simulink model "DP_CFGOC_SSP"  (R2023b)
settings: Solver=ode45  StartTime=0.0  StopTime=300  RelTol=1e-3  EnableMultiTasking=on
undefined symbols (not defined in the file): Als, Ats, D, G, Loa, MA, MRB, pa, Ta_p, Ta_x, Ta_y
libraries: mssSimulink x8, simulink x8, simulink_extras x5, fuzblock x3, marine_gnc x3
settings Model: Creator=Lenovo  LastModifiedBy=Ly Soi
settings SolverCC: AlgebraicLoopSolver=TrustRegion
settings DataIOCC: LimitDataPoints=on  SaveFormat=Array  SignalLoggingSaveFormat=ModelDataLogs  ReturnWorkspaceOutputs=off  SignalLoggingName=sigsOut
settings OptimizationCC: InitFltsAndDblsToZero=on  LifeSpan=inf
settings DebuggingCC: SaveWithParameterizedLinksMsg=none  UnderspecifiedInitializationDetection=Classic  MergeDetectMultiDrivingBlocksExec=none  SignalResolutionControl=TryResolveAllWithWarning  MultiTaskDSMMsg=warning  MultiTaskCondExecSysMsg=none  FcnCallInpInsideContextMsg=warning  UnconnectedInputMsg=warning  UnconnectedOutputMsg=warning  UnconnectedLineMsg=warning  SFUnexpectedBacktrackingDiag=warning  SFNoUnconditionalDefaultTransitionDiag=warning  ArithmeticOperatorsInVariantConditions=warning
settings HardwareCC: ProdBitPerPointer=32  ProdBitPerSizeT=32  ProdBitPerPtrDiffT=32  ProdLargestAtomicFloat=None  ProdIntDivRoundTo=Undefined  ProdEndianess=Unspecified  ProdWordSize=32  ProdHWDeviceType=32-bit Generic  TargetUnknown=on
settings ModelReferenceCC: EnableRefExpFcnMdlSchedulingChecks=on  PropagateSignalLabelsOutOfModel=off
settings SFSimCC: SimUseLocalCustomCode=off  CustomCodeUndefinedFunction=UseInterfaceOnly
settings RTWCC: RTWUseLocalCustomCode=off
settings CodeAppCC: StateflowObjectComments=on
settings GRTTargetCC: TargetFcnLib=ansi_tfl_tmw.mat  TargetLangStandard=C89/C90 (ANSI)  ModelReferenceCompliant=off  CombineOutputUpdateFcns=off  MatFileLogging=off  GRTInterface=on
settings ConfigComp: CovMetricSettings=dw  CovSaveCumulativeToWorkspaceVar=on  CovSaveSingleToWorkspaceVar=on  CovExternalEMLEnable=off  CovSFcnEnable=off

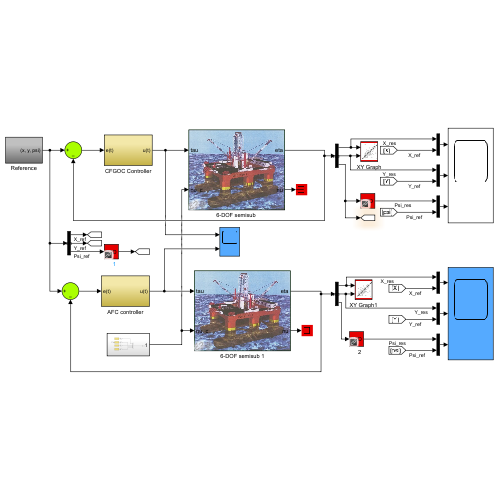
[thumbnail: Simulink's stored preview of the top-level diagram]
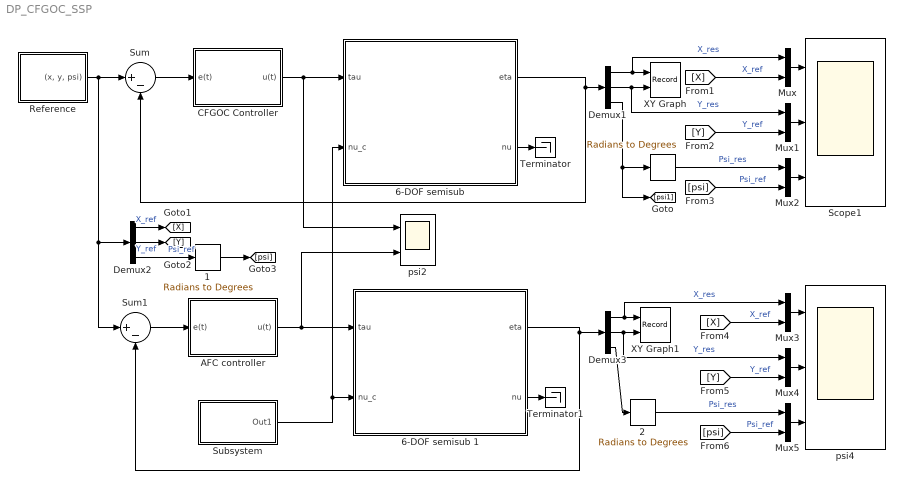
== system DP_CFGOC_SSP ==
  "    " : simulink_extras/Transformations/Radians to Degrees
  "    1" : simulink_extras/Transformations/Radians to Degrees
  "    2" : simulink_extras/Transformations/Radians to Degrees
  "6-DOF semisub " : Subsystem  AncestorBlock=mssSimulink/Marine craft models/6-DOF semisub  InitFcn=load MSS/VESSELS/rigModel/rig.mat  mask(6-DOF semisub){D=D, G=G, MA=MA, MRB=MRB}
      mask prompts: D "Linear damping matrix: D"; G "Spring matrix G:"; MA "System inertia added mass matrix: M"; MRB "System inertia rigid-body matrix"
      mask help:
      | Semisub low-speed model for DP.
      |
      | Inputs:
      |
      |    tau = 6 DOF control input vector (generalized force)
      |
      | Outputs:
      |
      |    eta = [x, y, z, phi, theta, psi]'
      |    nu  = [u, v, w, p, q, r]'
      mask Display:
      | image(imread('SIMULINK/figs/semisub.jpg'))
      | color('black'); port_label('output', 1, 'eta')
      | color('black'); port_label('output', 2, 'nu')
      | color('black'); port_label('input', 1, 'tau')
      | color('black'); port_label('input', 2, 'nu_c')
  6-DOF semisub 1 : Subsystem  AncestorBlock=mssSimulink/Marine craft models/6-DOF semisub  InitFcn=load MSS/VESSELS/rigModel/rig.mat  mask(6-DOF semisub){D=D, G=G, MA=MA, MRB=MRB}
      mask prompts: D "Linear damping matrix: D"; G "Spring matrix G:"; MA "System inertia added mass matrix: M"; MRB "System inertia rigid-body matrix"
      mask help:
      | Semisub low-speed model for DP.
      |
      | Inputs:
      |
      |    tau = 6 DOF control input vector (generalized force)
      |
      | Outputs:
      |
      |    eta = [x, y, z, phi, theta, psi]'
      |    nu  = [u, v, w, p, q, r]'
      mask Display:
      | image(imread('SIMULINK/figs/semisub.jpg'))
      | color('black'); port_label('output', 1, 'eta')
      | color('black'); port_label('output', 2, 'nu')
      | color('black'); port_label('input', 1, 'tau')
      | color('black'); port_label('input', 2, 'nu_c')
  AFC controller : Subsystem
  CFGOC Controller : Subsystem
  Demux1 : Demux  Outputs=3
      settings: DisplayOption=none
  Demux2 : Demux  Outputs=3
      settings: DisplayOption=none
  Demux3 : Demux  Outputs=3
      settings: DisplayOption=none
  Mux{,1..5} (6 alike) : Mux  Inputs=2
  Reference : Subsystem
  Scope1 : Scope  NumInputPorts=3
  Subsystem : Subsystem
  Sum : Sum  Inputs=|+-
  Sum1 : Sum  Inputs=|+-
  Terminator : Terminator
  Terminator1 : Terminator
  XY Graph : Record  FileSettingsInternal="{\"entries\":[{\"content\":{\"excelSettings\":{\"content\":{},\"type\":\"Streamout.ExcelSettings\"}},\"type\":\"Streamout.FileSettingStorage\",\"uuid\":\"\"}],\"packageUris\":[\"http:\\/\\/schema.mathworks.com\\/mf0\\/streamout_blocks\\/R2020a\"],\"version\":\"1.0\"}"  Layout=[1 1]  SignalsInternal="{\"entries\":[{\"content\":{\"signals\":[{\"content\":{\"blockPath\":[],\"dimensions\":[1],\"domain\":\"\",\"lineColor\":\"#a2142f\",\"plots\":[1],\"port\":1,\"signalID\":43,\"signalName\":\"XY Graph:1\"},\"type\":\"RecordBlkView.Signal\",\"uuid\":\"\"},{\"content\":{\"blockPath\":[],\"dimensions\":[1],\"domain\":\"\",\"lineColor\":\"#139fff\",\"plots\":[1],\"port\":2,\"signalID\":46,\"signalName\":\"XY Graph:2\"},\"type\":\"RecordBlkView.Signal\",\"uuid\":\"\"}]},\"type\":\"RecordBlkView.InputSignals\",\"uuid\":\"\"}],\"packageUris\":[\"http:\\/\\/schema.mathworks.com\\/mf0\\/streamout_blocks\\/R2020a\"],\"version\":\"1.0\"}"  VisualizationBindings="{\"xyplotplugin\":{\"info\":[{\"series\":[{\"bindingParametersList\":[{\"parameter\":\"X-Axis\",\"signalID\":43,\"signalName\":\"XY Graph:1\"},{\"parameter\":\"Y-Axis\",\"signalID\":46,\"signalName\":\"XY Graph:2\"}],\"seriesID\":58743}],\"subplotID\":1}]}}"  CompatibilityTag=XY  st=0.1
  XY Graph1 : Record  FileSettingsInternal="{\"entries\":[{\"content\":{\"excelSettings\":{\"content\":{},\"type\":\"Streamout.ExcelSettings\"}},\"type\":\"Streamout.FileSettingStorage\",\"uuid\":\"\"}],\"packageUris\":[\"http:\\/\\/schema.mathworks.com\\/mf0\\/streamout_blocks\\/R2020a\"],\"version\":\"1.0\"}"  Layout=[1 1]  SignalsInternal="{\"entries\":[{\"content\":{\"signals\":[{\"content\":{\"blockPath\":[],\"dimensions\":[1],\"domain\":\"\",\"lineColor\":\"#a2142f\",\"plots\":[1],\"port\":1,\"signalID\":35,\"signalName\":\"X_res\"},\"type\":\"RecordBlkView.Signal\",\"uuid\":\"\"},{\"content\":{\"blockPath\":[],\"dimensions\":[1],\"domain\":\"\",\"lineColor\":\"#139fff\",\"plots\":[1],\"port\":2,\"signalID\":38,\"signalName\":\"Y_res\"},\"type\":\"RecordBlkView.Signal\",\"uuid\":\"\"}]},\"type\":\"RecordBlkView.InputSignals\",\"uuid\":\"\"}],\"packageUris\":[\"http:\\/\\/schema.mathworks.com\\/mf0\\/streamout_blocks\\/R2020a\"],\"version\":\"1.0\"}"  VisualizationBindings="{\"xyplotplugin\":{\"info\":[{\"series\":[{\"bindingParametersList\":[{\"parameter\":\"X-Axis\",\"signalID\":35,\"signalName\":\"X_res\"},{\"parameter\":\"Y-Axis\",\"signalID\":38,\"signalName\":\"Y_res\"}],\"seriesID\":17634}],\"subplotID\":1}]}}"  CompatibilityTag=XY  st=0.1
  psi2 : Scope  NumInputPorts=2
  psi4 : Scope  NumInputPorts=3
  wires:
  Sum/1 -> CFGOC Controller/1(e(t))
  "6-DOF semisub "/2(nu) -> Terminator/1
  Demux1/1 -> XY Graph/1, Mux/1  "X_res"
  Demux1/2 -> XY Graph/2, Mux1/1  "Y_res"
  "6-DOF semisub "/1(eta) -> Sum/2, Demux1/1
  Demux1/3 -> "    "/1, [psi1]
  Mux/1 -> Scope1/1
  [X] -> Mux/2  "X_ref"
  Mux1/1 -> Scope1/2
  [Y] -> Mux1/2  "Y_ref"
  Mux2/1 -> Scope1/3
  [psi] -> Mux2/2  "Psi_ref"
  "    "/1 -> Mux2/1  "Psi_res"
  "    1"/1 -> [psi]
  Reference/1("(x, y, psi)") -> Sum1/1, Demux2/1, Sum/1
  Sum1/1 -> AFC controller/1(e(t))
  6-DOF semisub 1/2(nu) -> Terminator1/1
  Demux3/1 -> XY Graph1/1, Mux3/1  "X_res"
  Demux3/2 -> XY Graph1/2, Mux4/1  "Y_res"
  6-DOF semisub 1/1(eta) -> Sum1/2, Demux3/1
  Demux3/3 -> "    2"/1
  Mux3/1 -> psi4/1
  Demux2/1 -> [X]  "X_ref"
  Mux4/1 -> psi4/2
  Demux2/2 -> [Y]  "Y_ref"
  Mux5/1 -> psi4/3
  Demux2/3 -> "    1"/1  "Psi_ref"
  "    2"/1 -> Mux5/1  "Psi_res"
  [X] -> Mux3/2  "X_ref"
  [Y] -> Mux4/2  "Y_ref"
  [psi] -> Mux5/2  "Psi_ref"
  Subsystem/1(Out1) -> 6-DOF semisub 1/2(nu_c), "6-DOF semisub "/2(nu_c)
  CFGOC Controller/1(u(t)) -> psi2/1, "6-DOF semisub "/1(tau)
  AFC controller/1(u(t)) -> psi2/2, 6-DOF semisub 1/1(tau)

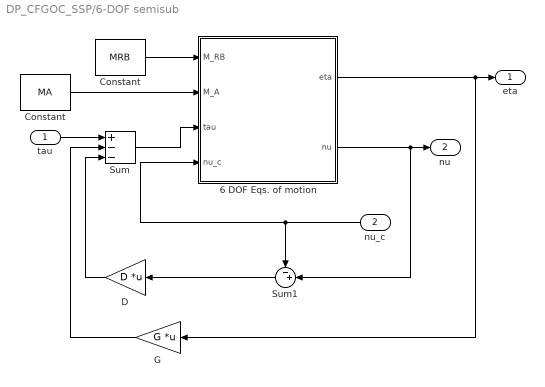
== system DP_CFGOC_SSP/6-DOF semisub  ==
  tau : Inport
  nu_c : Inport  Port=2
  "6 DOF Eqs. of motion " : Subsystem  AncestorBlock=mssSimulink/Modelling/Kinetics /6 DOF Eqs. of motion  mask(Equations of motion){CoriolisOnOff=on, nu0=[0 0 0 0 0 0], eta0=[0 0 0 0 0 0]}
      mask prompts: CoriolisOnOff "Coriolis and centripetal forces (check box to turn on)"; nu0 "Initial velocities (u,v,w,p,q,r)"; eta0 "Initial position/attitude (x,y,z,phi,theta,psi)"
      mask help:
      | 6 DOF equations of motion (surge, sway, heave, roll, pitch and yaw)
      |
      |    eta_dot = J(eta)*nu
      |    (M_RB+M_A)*nu_dot + C_RB(nu)nu+C_A(nu_r)nu_r  =  tau
      |
      |    nu_r = nu-nu_c    (relative velocity)
      |    nu_c = [u_c,v_c,w_c,0,0,0]  slowly-varying current velocity
      |
      | where nu = [u,v,w,p,q,r]'  and eta = [x,y,x,phi,theta,psi]'
      |
      | The Coriolis and centripetal matrix C(nu) is computed automatically using the system inertia matrix M and nu,  see Chapter 3 in Fossen (2002) for details.
      |
      | T. I. Fossen (2002). Marine Control Systems: Guidance, Navigation and Control of Ships, Rigs and Underwater Vehicles, Marine Cybernetics AS, ISBN 82-92356-00-2
  Constant : Constant  Value=MRB
  "Constant " : Constant  Value=MA
  D : Gain  Gain=D  Multiplication=Matrix(K*u)  SaturateOnIntegerOverflow=on  OutDataTypeStr=Inherit: Same as input  ParamDataTypeStr=Inherit: Same as input
  G : Gain  Gain=G  Multiplication=Matrix(K*u)  SaturateOnIntegerOverflow=on  OutDataTypeStr=Inherit: Same as input  ParamDataTypeStr=Inherit: Same as input
  Sum : Sum  Inputs=+--  InputSameDT=on  SaturateOnIntegerOverflow=on  OutDataTypeStr=Inherit: Same as first input
  Sum1 : Sum  Inputs=-+|  SaturateOnIntegerOverflow=on
  eta : Outport  InitialOutput=0  VectorParamsAs1DForOutWhenUnconnected=off
  nu : Outport  Port=2  InitialOutput=0  VectorParamsAs1DForOutWhenUnconnected=off
  wires:
  tau/1 -> Sum/1
  D/1 -> Sum/3
  G/1 -> Sum/2
  "6 DOF Eqs. of motion "/2(nu) -> Sum1/2, nu/1
  "6 DOF Eqs. of motion "/1(eta) -> eta/1, G/1
  Constant/1 -> "6 DOF Eqs. of motion "/1(M_RB)
  nu_c/1 -> Sum1/1, "6 DOF Eqs. of motion "/4(nu_c)
  Sum1/1 -> D/1
  Sum/1 -> "6 DOF Eqs. of motion "/3(tau)
  "Constant "/1 -> "6 DOF Eqs. of motion "/2(M_A)

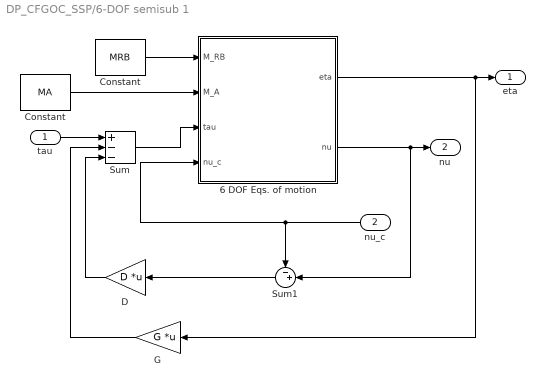
== system DP_CFGOC_SSP/6-DOF semisub 1 ==
  tau : Inport
  nu_c : Inport  Port=2
  "6 DOF Eqs. of motion " : Subsystem  AncestorBlock=mssSimulink/Modelling/Kinetics /6 DOF Eqs. of motion  mask(Equations of motion){CoriolisOnOff=on, nu0=[0 0 0 0 0 0], eta0=[0 0 0 0 0 0]}
      mask prompts: CoriolisOnOff "Coriolis and centripetal forces (check box to turn on)"; nu0 "Initial velocities (u,v,w,p,q,r)"; eta0 "Initial position/attitude (x,y,z,phi,theta,psi)"
      mask help:
      | 6 DOF equations of motion (surge, sway, heave, roll, pitch and yaw)
      |
      |    eta_dot = J(eta)*nu
      |    (M_RB+M_A)*nu_dot + C_RB(nu)nu+C_A(nu_r)nu_r  =  tau
      |
      |    nu_r = nu-nu_c    (relative velocity)
      |    nu_c = [u_c,v_c,w_c,0,0,0]  slowly-varying current velocity
      |
      | where nu = [u,v,w,p,q,r]'  and eta = [x,y,x,phi,theta,psi]'
      |
      | The Coriolis and centripetal matrix C(nu) is computed automatically using the system inertia matrix M and nu,  see Chapter 3 in Fossen (2002) for details.
      |
      | T. I. Fossen (2002). Marine Control Systems: Guidance, Navigation and Control of Ships, Rigs and Underwater Vehicles, Marine Cybernetics AS, ISBN 82-92356-00-2
  Constant : Constant  Value=MRB
  "Constant " : Constant  Value=MA
  D : Gain  Gain=D  Multiplication=Matrix(K*u)  SaturateOnIntegerOverflow=on  OutDataTypeStr=Inherit: Same as input  ParamDataTypeStr=Inherit: Same as input
  G : Gain  Gain=G  Multiplication=Matrix(K*u)  SaturateOnIntegerOverflow=on  OutDataTypeStr=Inherit: Same as input  ParamDataTypeStr=Inherit: Same as input
  Sum : Sum  Inputs=+--  InputSameDT=on  SaturateOnIntegerOverflow=on  OutDataTypeStr=Inherit: Same as first input
  Sum1 : Sum  Inputs=-+|  SaturateOnIntegerOverflow=on
  eta : Outport  InitialOutput=0  VectorParamsAs1DForOutWhenUnconnected=off
  nu : Outport  Port=2  InitialOutput=0  VectorParamsAs1DForOutWhenUnconnected=off
  wires:
  tau/1 -> Sum/1
  D/1 -> Sum/3
  G/1 -> Sum/2
  "6 DOF Eqs. of motion "/2(nu) -> Sum1/2, nu/1
  "6 DOF Eqs. of motion "/1(eta) -> eta/1, G/1
  Constant/1 -> "6 DOF Eqs. of motion "/1(M_RB)
  nu_c/1 -> Sum1/1, "6 DOF Eqs. of motion "/4(nu_c)
  Sum1/1 -> D/1
  Sum/1 -> "6 DOF Eqs. of motion "/3(tau)
  "Constant "/1 -> "6 DOF Eqs. of motion "/2(M_A)

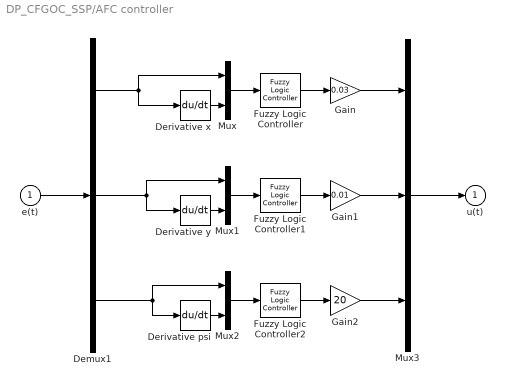
== system DP_CFGOC_SSP/AFC controller ==
  e(t) : Inport
  Demux1 : Demux  Outputs=3
  Derivative psi : Derivative
  Derivative x : Derivative
  Derivative y : Derivative
  Fuzzy Logic Controller : fuzblock/Fuzzy Logic  Controller  FIS='motau1moi.fis'  OutputSampleNumber=101  DataType=double  FuzzifiedInputs=off  RuleFiringStrengths=off  RuleOutputs=off  AggregatedOutputs=off  SimulateUsing=Interpreted execution  OutOfRangeInputValueMessage=warning  NoRuleFiredMessage=warning  EmptyOutputFuzzySetMessage=warning
  Fuzzy Logic Controller1 : fuzblock/Fuzzy Logic  Controller  FIS='motau2moi.fis'  OutputSampleNumber=101  DataType=double  FuzzifiedInputs=off  RuleFiringStrengths=off  RuleOutputs=off  AggregatedOutputs=off  SimulateUsing=Interpreted execution  OutOfRangeInputValueMessage=warning  NoRuleFiredMessage=warning  EmptyOutputFuzzySetMessage=warning
  Fuzzy Logic Controller2 : fuzblock/Fuzzy Logic  Controller  FIS='motau3moi.fis'  OutputSampleNumber=101  DataType=double  FuzzifiedInputs=off  RuleFiringStrengths=off  RuleOutputs=off  AggregatedOutputs=off  SimulateUsing=Interpreted execution  OutOfRangeInputValueMessage=warning  NoRuleFiredMessage=warning  EmptyOutputFuzzySetMessage=warning
  Gain : Gain  Gain=0.03
  Gain1 : Gain  Gain=0.01
  Gain2 : Gain  Gain=20
  Mux : Mux  Inputs=2
  Mux1 : Mux  Inputs=2
  Mux2 : Mux  Inputs=2
  Mux3 : Mux  Inputs=3
  u(t) : Outport
  wires:
  Mux3/1 -> u(t)/1
  e(t)/1 -> Demux1/1
  Gain1/1 -> Mux3/2
  Gain2/1 -> Mux3/3
  Fuzzy Logic Controller/1 -> Gain/1
  Gain/1 -> Mux3/1
  Fuzzy Logic Controller2/1 -> Gain2/1
  Fuzzy Logic Controller1/1 -> Gain1/1
  Demux1/1 -> Mux/1, Derivative x/1
  Demux1/2 -> Derivative y/1, Mux1/1
  Demux1/3 -> Derivative psi/1, Mux2/1
  Derivative y/1 -> Mux1/2
  Derivative x/1 -> Mux/2
  Derivative psi/1 -> Mux2/2
  Mux/1 -> Fuzzy Logic Controller/1
  Mux1/1 -> Fuzzy Logic Controller1/1
  Mux2/1 -> Fuzzy Logic Controller2/1

== system DP_CFGOC_SSP/CFGOC Controller ==
  e(t) : Inport
  Demux1 : Demux  Outputs=3
  GA-Psi : Subsystem
  GA-X : Subsystem
  GA-Y : Subsystem
  Gain : Gain  Gain=0.3
  Gain1 : Gain  Gain=0.3
  Gain2 : Gain
  Mux3 : Mux  Inputs=3
  u(t) : Outport
  wires:
  Mux3/1 -> u(t)/1
  Demux1/2 -> GA-Y/1(e_h)
  Demux1/3 -> GA-Psi/1(e_h)
  e(t)/1 -> Demux1/1
  Gain1/1 -> Mux3/2
  Gain2/1 -> Mux3/3
  GA-X/1(u_h) -> Gain/1
  Demux1/1 -> GA-X/1(e_h)
  Gain/1 -> Mux3/1
  GA-Psi/1(u_h) -> Gain2/1
  GA-Y/1(u_h) -> Gain1/1

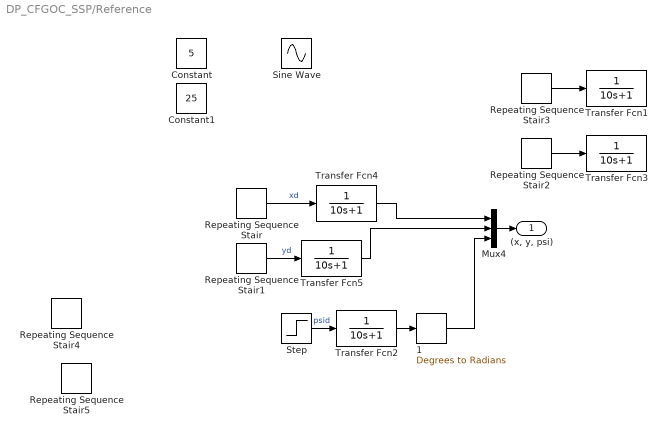
== system DP_CFGOC_SSP/Reference ==
  "     1" : simulink_extras/Transformations/Degrees to Radians
  Constant : Constant  Value=5
  Constant1 : Constant  Value=25
  Mux4 : Mux  Inputs=3
  Repeating Sequence Stair : simulink/Sources/Repeating Sequence Stair  OutValues=[10 0 10]  tsamp=100  OutMin=[]  OutMax=[]  OutDataTypeStr=double  OutputDataTypeScalingMode=double  OutDataType=fixdt(0,8)  ConRadixGroup=Best Precision: Vector-wise  OutScaling=2^-12
  Repeating Sequence Stair1 : simulink/Sources/Repeating Sequence Stair  OutValues=[0 10 10]  tsamp=100  OutMin=[]  OutMax=[]  OutDataTypeStr=double  OutputDataTypeScalingMode=double  OutDataType=fixdt(0,8)  ConRadixGroup=Best Precision: Vector-wise  OutScaling=2^-12
  Repeating Sequence Stair2 : simulink/Sources/Repeating Sequence Stair  OutValues=[7 -7 0 7]  tsamp=10  OutMin=[]  OutMax=[]  OutDataTypeStr=double  OutputDataTypeScalingMode=double  OutDataType=fixdt(0,8)  ConRadixGroup=Best Precision: Vector-wise  OutScaling=2^-12
  Repeating Sequence Stair3 : simulink/Sources/Repeating Sequence Stair  OutValues=[-7 7 0 7]  tsamp=10  OutMin=[]  OutMax=[]  OutDataTypeStr=double  OutputDataTypeScalingMode=double  OutDataType=fixdt(0,8)  ConRadixGroup=Best Precision: Vector-wise  OutScaling=2^-12
  Repeating Sequence Stair4 : simulink/Sources/Repeating Sequence Stair  OutValues="[0\t0\t0\t0\t0\t0\t0\t0\t0\t0\t0\t0\t0\t0\t0\t0\t0\t0\t0\t0\t0\t0\t0\t0\t0\t0\t0\t0\t0\t0\t0\t0\t0\t0\t0\t0\t0\t0\t0\t0\t0\t0\t0\t0\t0\t0\t0\t0\t0\t0\t0\t0\t0\t0\t0\t0\t0\t0\t0\t0\t0\t0\t0\t0\t0\t0\t0\t0\t0\t0\t0\t0\t0\t0\t0\t0\t0\t0\t0\t0\t0\t0\t0\t0\t0\t0\t0\t0\t0\t0\t0\t0\t0\t0\t0\t0\t0\t0\t0\t0\t0\t0\t0\t0.2\t0.4\t0.6\t0.8\t1\t1.2\t1.4\t1.6\t1.8\t2\t2.2\t2.4\t2.6\t2.8\t3\t3.2\t3.4\t3.6\t3.8\t4\t4.2\t4.4\t4.6\t4.8\t5\t5.2\t5.4\t5.6\t5.8\t6\t6.2\t6.4\t6.6\t6.8\t7\t7.2\t7.4\t7.6\t7.8\t8\t8.2\t8.4\t8.6\t8.8\t9\t9.2\t9.4\t9.6\t9.8\t10\t10\t10\t10\t10\t10\t10\t10\t10\t10\t10\t10\t10\t10\t10\t10\t10\t10\t10\t10\t10\t10\t10\t10\t10\t10\t10\t10\t10\t10\t10\t10\t10\t10\t10\t10\t10\t10\t10\t10\t10\t10\t10\t10\t10\t10\t10\t10\t10\t10\t10\t10]"  tsamp=1  OutMin=[]  OutMax=[]  OutDataTypeStr=double  OutputDataTypeScalingMode=double  OutDataType=fixdt(0,8)  ConRadixGroup=Best Precision: Vector-wise  OutScaling=2^-12
  Repeating Sequence Stair5 : simulink/Sources/Repeating Sequence Stair  OutValues="[0\t0.2\t0.4\t0.6\t0.8\t1\t1.2\t1.4\t1.6\t1.8\t2\t2.2\t2.4\t2.6\t2.8\t3\t3.2\t3.4\t3.6\t3.8\t4\t4.2\t4.4\t4.6\t4.8\t5\t5.2\t5.4\t5.6\t5.8\t6\t6.2\t6.4\t6.6\t6.8\t7\t7.2\t7.4\t7.6\t7.8\t8\t8.2\t8.4\t8.6\t8.8\t9\t9.2\t9.4\t9.6\t9.8\t10\t10\t10\t10\t10\t10\t10\t10\t10\t10\t10\t10\t10\t10\t10\t10\t10\t10\t10\t10\t10\t10\t10\t10\t10\t10\t10\t10\t10\t10\t10\t10\t10\t10\t10\t10\t10\t10\t10\t10\t10\t10\t10\t10\t10\t10\t10\t10\t10\t10\t10\t10\t10\t10\t10\t10\t10\t10\t10\t10\t10\t10\t10\t10\t10\t10\t10\t10\t10\t10\t10\t10\t10\t10\t10\t10\t10\t10\t10\t10\t10\t10\t10\t10\t10\t10\t10\t10\t10\t10\t10\t10\t10\t10\t10\t10\t10\t10\t10\t10\t10\t10\t10\t10\t10\t10\t10\t10\t10\t10\t10\t10\t10\t10\t10\t10\t10\t10\t10\t10\t10\t10\t10\t10\t10\t10\t10\t10\t10\t10\t10\t10\t10\t10\t10\t10\t10\t10\t10\t10\t10\t10\t10\t10\t10\t10\t10\t10\t10\t10\t10\t10\t10\t10]"  tsamp=1  OutMin=[]  OutMax=[]  OutDataTypeStr=double  OutputDataTypeScalingMode=double  OutDataType=fixdt(0,8)  ConRadixGroup=Best Precision: Vector-wise  OutScaling=2^-12
  Sine Wave : Sin  Frequency=4  SampleTime=0
  Step : Step  Time=0  After=20  SampleTime=0
  Transfer Fcn{1..5} (5 alike) : TransferFcn  Denominator=[10 1]
  "(x, y, psi)" : Outport
  wires:
  Mux4/1 -> "(x, y, psi)"/1
  "     1"/1 -> Mux4/3
  Step/1 -> Transfer Fcn2/1  "psid"
  Transfer Fcn2/1 -> "     1"/1
  Repeating Sequence Stair2/1 -> Transfer Fcn3/1
  Repeating Sequence Stair3/1 -> Transfer Fcn1/1
  Repeating Sequence Stair/1 -> Transfer Fcn4/1  "xd"
  Repeating Sequence Stair1/1 -> Transfer Fcn5/1  "yd"
  Transfer Fcn4/1 -> Mux4/1
  Transfer Fcn5/1 -> Mux4/2

== system DP_CFGOC_SSP/Subsystem ==
  Current impact : Subsystem
  Mux : Mux
  Noise impact : Subsystem
  Wave impact : Subsystem
  Wind impact : Subsystem
  adjust_Noi : Gain
  adjust_c : Gain
  adjust_w : Gain  Gain=2
  adjust_wi : Gain
  Out1 : Outport
  wires:
  Wave impact/1(Tau_wave) -> adjust_w/1
  Current impact/1(Tau_current) -> adjust_c/1
  [psi1] -> Wind impact/1(psi)
  Noise impact/1(Tau_Noise) -> adjust_Noi/1
  Wind impact/1(Tau_wind) -> adjust_wi/1
  adjust_wi/1 -> Mux/2
  adjust_w/1 -> Mux/1
  adjust_c/1 -> Mux/3
  adjust_Noi/1 -> Mux/4
  Mux/1 -> Out1/1

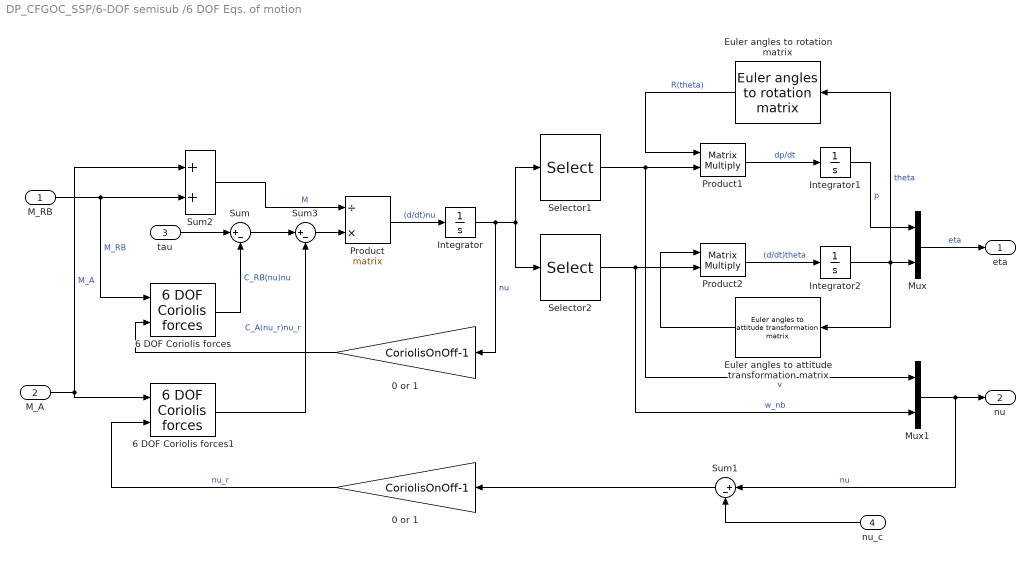
== system DP_CFGOC_SSP/6-DOF semisub /6 DOF Eqs. of motion  ==
  M_RB : Inport
  M_A : Inport  Port=2
  tau : Inport  Port=3
  nu_c : Inport  Port=4
  0 or 1 : Gain  Gain=CoriolisOnOff-1  SaturateOnIntegerOverflow=on  OutDataTypeStr=Inherit: Same as input  ParamDataTypeStr=Inherit: Same as input
  "0 or 1   " : Gain  Gain=CoriolisOnOff-1  SaturateOnIntegerOverflow=on  OutDataTypeStr=Inherit: Same as input  ParamDataTypeStr=Inherit: Same as input
  6 DOF Coriolis forces : mssSimulink/Modelling/Kinetics /Support/6 DOF Coriolis forces  SystemSampleTime=-1  VariantActivationTime=update diagram  AllowFlexibleInterface=on  Latency=0  AutoFrameSizeCalculation=off
  6 DOF Coriolis forces1 : mssSimulink/Modelling/Kinetics /Support/6 DOF Coriolis forces  SystemSampleTime=-1  VariantActivationTime=update diagram  AllowFlexibleInterface=on  Latency=0  AutoFrameSizeCalculation=off
  Euler angles to rotation matrix : mssSimulink/Modelling/Kinematics/Euler angles to rotation matrix
  Euler angles to attitude transformation matrix : mssSimulink/Modelling/Kinematics/Euler angles to attitude transformation matrix
  Integrator : Integrator  InitialCondition=nu0
  Integrator1 : Integrator  InitialCondition=eta0(1:3)
  Integrator2 : Integrator  InitialCondition=eta0(4:6)
  Mux : Mux  Inputs=2
  Mux1 : Mux  Inputs=2
  Product : Product  Inputs=/*  Multiplication=Matrix(*)  SaturateOnIntegerOverflow=on  OutDataTypeStr=Inherit: Same as first input
  Product1 : Product  Inputs=**  Multiplication=Matrix(*)  SaturateOnIntegerOverflow=on  OutDataTypeStr=Inherit: Same as first input
  Product2 : Product  Inputs=**  Multiplication=Matrix(*)  SaturateOnIntegerOverflow=on  OutDataTypeStr=Inherit: Same as first input
  Selector1 : Selector  InputPortWidth=6  IndexOptions=Index vector (dialog)  Indices=[1 2 3]  OutputSizes=1
  Selector2 : Selector  InputPortWidth=6  IndexOptions=Index vector (dialog)  Indices=[4 5 6]  OutputSizes=1
  Sum : Sum  Inputs=|+-  SaturateOnIntegerOverflow=on
  Sum1 : Sum  Inputs=|+-  SaturateOnIntegerOverflow=on
  Sum2 : Sum  SaturateOnIntegerOverflow=on
  Sum3 : Sum  Inputs=|+-  SaturateOnIntegerOverflow=on
  eta : Outport  VectorParamsAs1DForOutWhenUnconnected=off
  nu : Outport  Port=2  VectorParamsAs1DForOutWhenUnconnected=off
  wires:
  0 or 1/1 -> 6 DOF Coriolis forces/2
  6 DOF Coriolis forces/1 -> Sum/2  "C_RB(nu)nu"
  tau/1 -> Sum/1
  Euler angles to attitude transformation matrix/1 -> Product2/1
  Mux1/1 -> Sum1/1, nu/1  "nu"
  Mux/1 -> eta/1  "eta"
  Integrator1/1 -> Mux/1  "p"
  Integrator2/1 -> Euler angles to attitude transformation matrix/1, Euler angles to rotation matrix/1, Mux/2  "theta"
  Product2/1 -> Integrator2/1  "(d/dt)theta"
  Euler angles to rotation matrix/1 -> Product1/1  "R(theta)"
  Product1/1 -> Integrator1/1  "dp/dt"
  Selector2/1 -> Product2/2, Mux1/2  "w_nb"
  Selector1/1 -> Mux1/1, Product1/2  "v"
  Integrator/1 -> 0 or 1/1, Selector2/1, Selector1/1  "nu"
  Product/1 -> Integrator/1  "(d/dt)nu"
  M_RB/1 -> 6 DOF Coriolis forces/1, Sum2/2  "M_RB"
  M_A/1 -> 6 DOF Coriolis forces1/1, Sum2/1  "M_A"
  Sum2/1 -> Product/1  "M"
  Sum/1 -> Sum3/1
  Sum3/1 -> Product/2
  6 DOF Coriolis forces1/1 -> Sum3/2  "C_A(nu_r)nu_r"
  "0 or 1   "/1 -> 6 DOF Coriolis forces1/2  "nu_r"
  Sum1/1 -> "0 or 1   "/1
  nu_c/1 -> Sum1/2

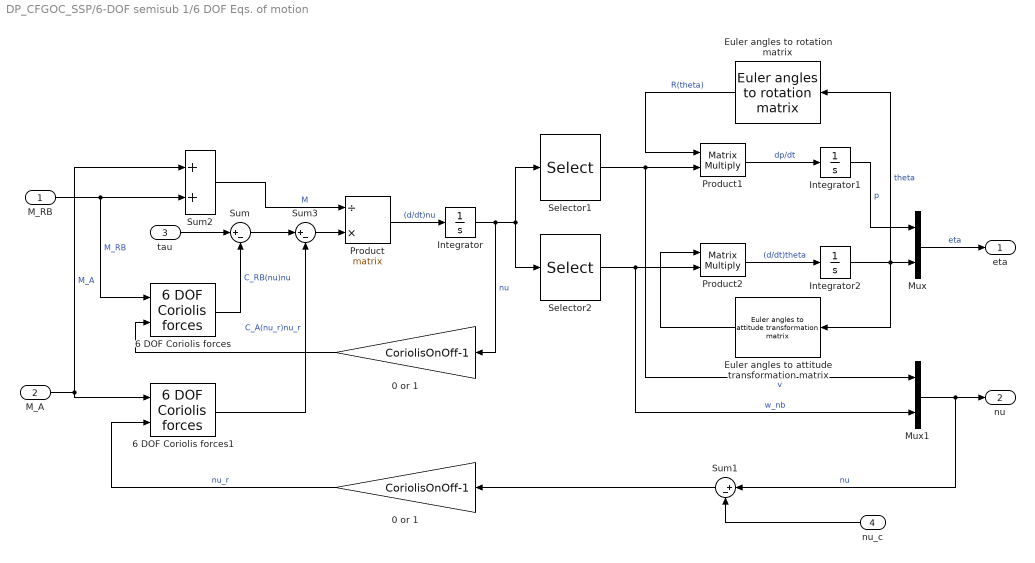
== system DP_CFGOC_SSP/6-DOF semisub 1/6 DOF Eqs. of motion  ==
  M_RB : Inport
  M_A : Inport  Port=2
  tau : Inport  Port=3
  nu_c : Inport  Port=4
  0 or 1 : Gain  Gain=CoriolisOnOff-1  SaturateOnIntegerOverflow=on  OutDataTypeStr=Inherit: Same as input  ParamDataTypeStr=Inherit: Same as input
  "0 or 1   " : Gain  Gain=CoriolisOnOff-1  SaturateOnIntegerOverflow=on  OutDataTypeStr=Inherit: Same as input  ParamDataTypeStr=Inherit: Same as input
  6 DOF Coriolis forces : mssSimulink/Modelling/Kinetics /Support/6 DOF Coriolis forces  SystemSampleTime=-1  VariantActivationTime=update diagram  AllowFlexibleInterface=on  Latency=0  AutoFrameSizeCalculation=off
  6 DOF Coriolis forces1 : mssSimulink/Modelling/Kinetics /Support/6 DOF Coriolis forces  SystemSampleTime=-1  VariantActivationTime=update diagram  AllowFlexibleInterface=on  Latency=0  AutoFrameSizeCalculation=off
  Euler angles to rotation matrix : mssSimulink/Modelling/Kinematics/Euler angles to rotation matrix
  Euler angles to attitude transformation matrix : mssSimulink/Modelling/Kinematics/Euler angles to attitude transformation matrix
  Integrator : Integrator  InitialCondition=nu0
  Integrator1 : Integrator  InitialCondition=eta0(1:3)
  Integrator2 : Integrator  InitialCondition=eta0(4:6)
  Mux : Mux  Inputs=2
  Mux1 : Mux  Inputs=2
  Product : Product  Inputs=/*  Multiplication=Matrix(*)  SaturateOnIntegerOverflow=on  OutDataTypeStr=Inherit: Same as first input
  Product1 : Product  Inputs=**  Multiplication=Matrix(*)  SaturateOnIntegerOverflow=on  OutDataTypeStr=Inherit: Same as first input
  Product2 : Product  Inputs=**  Multiplication=Matrix(*)  SaturateOnIntegerOverflow=on  OutDataTypeStr=Inherit: Same as first input
  Selector1 : Selector  InputPortWidth=6  IndexOptions=Index vector (dialog)  Indices=[1 2 3]  OutputSizes=1
  Selector2 : Selector  InputPortWidth=6  IndexOptions=Index vector (dialog)  Indices=[4 5 6]  OutputSizes=1
  Sum : Sum  Inputs=|+-  SaturateOnIntegerOverflow=on
  Sum1 : Sum  Inputs=|+-  SaturateOnIntegerOverflow=on
  Sum2 : Sum  SaturateOnIntegerOverflow=on
  Sum3 : Sum  Inputs=|+-  SaturateOnIntegerOverflow=on
  eta : Outport  VectorParamsAs1DForOutWhenUnconnected=off
  nu : Outport  Port=2  VectorParamsAs1DForOutWhenUnconnected=off
  wires:
  0 or 1/1 -> 6 DOF Coriolis forces/2
  6 DOF Coriolis forces/1 -> Sum/2  "C_RB(nu)nu"
  tau/1 -> Sum/1
  Euler angles to attitude transformation matrix/1 -> Product2/1
  Mux1/1 -> Sum1/1, nu/1  "nu"
  Mux/1 -> eta/1  "eta"
  Integrator1/1 -> Mux/1  "p"
  Integrator2/1 -> Euler angles to attitude transformation matrix/1, Euler angles to rotation matrix/1, Mux/2  "theta"
  Product2/1 -> Integrator2/1  "(d/dt)theta"
  Euler angles to rotation matrix/1 -> Product1/1  "R(theta)"
  Product1/1 -> Integrator1/1  "dp/dt"
  Selector2/1 -> Product2/2, Mux1/2  "w_nb"
  Selector1/1 -> Mux1/1, Product1/2  "v"
  Integrator/1 -> 0 or 1/1, Selector2/1, Selector1/1  "nu"
  Product/1 -> Integrator/1  "(d/dt)nu"
  M_RB/1 -> 6 DOF Coriolis forces/1, Sum2/2  "M_RB"
  M_A/1 -> 6 DOF Coriolis forces1/1, Sum2/1  "M_A"
  Sum2/1 -> Product/1  "M"
  Sum/1 -> Sum3/1
  Sum3/1 -> Product/2
  6 DOF Coriolis forces1/1 -> Sum3/2  "C_A(nu_r)nu_r"
  "0 or 1   "/1 -> 6 DOF Coriolis forces1/2  "nu_r"
  Sum1/1 -> "0 or 1   "/1
  nu_c/1 -> Sum1/2

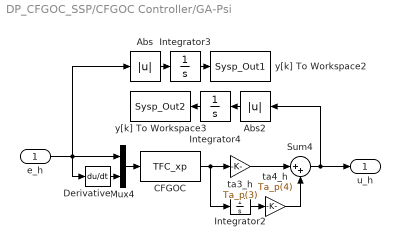
== system DP_CFGOC_SSP/CFGOC Controller/GA-Psi ==
  e_h : Inport
  Abs : Abs  SaturateOnIntegerOverflow=off
  Abs2 : Abs  SaturateOnIntegerOverflow=off
  CFGOC : MATLABFcn  MATLABFcn=TFC_xp  OutputDimensions=1
  Derivative : Derivative
  Integrator2 : Integrator
  Integrator3 : Integrator
  Integrator4 : Integrator
  Mux4 : Mux  Inputs=2
  Sum4 : Sum  Inputs=|++  InputSameDT=on  SaturateOnIntegerOverflow=on  OutDataTypeStr=Inherit: Same as first input
  ta3_h : Gain  Gain=Ta_p(3)
  ta4_h : Gain  Gain=Ta_p(4)
  y[k] To Workspace2 : ToWorkspace  VariableName=Sysp_Out1  SaveFormat=Timeseries  SampleTime=-1
  y[k] To Workspace3 : ToWorkspace  VariableName=Sysp_Out2  SaveFormat=Timeseries  SampleTime=-1
  u_h : Outport
  wires:
  Sum4/1 -> u_h/1, Abs2/1
  Derivative/1 -> Mux4/2
  Mux4/1 -> CFGOC/1
  CFGOC/1 -> ta3_h/1, Integrator2/1
  Integrator2/1 -> ta4_h/1
  ta4_h/1 -> Sum4/2
  ta3_h/1 -> Sum4/1
  e_h/1 -> Abs/1, Derivative/1, Mux4/1
  Integrator3/1 -> y[k] To Workspace2/1
  Integrator4/1 -> y[k] To Workspace3/1
  Abs/1 -> Integrator3/1
  Abs2/1 -> Integrator4/1

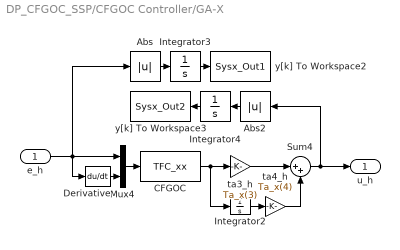
== system DP_CFGOC_SSP/CFGOC Controller/GA-X ==
  e_h : Inport
  Abs : Abs  SaturateOnIntegerOverflow=off
  Abs2 : Abs  SaturateOnIntegerOverflow=off
  CFGOC : MATLABFcn  MATLABFcn=TFC_xx  OutputDimensions=1
  Derivative : Derivative
  Integrator2 : Integrator
  Integrator3 : Integrator
  Integrator4 : Integrator
  Mux4 : Mux  Inputs=2
  Sum4 : Sum  Inputs=|++  InputSameDT=on  SaturateOnIntegerOverflow=on  OutDataTypeStr=Inherit: Same as first input
  ta3_h : Gain  Gain=Ta_x(3)
  ta4_h : Gain  Gain=Ta_x(4)
  y[k] To Workspace2 : ToWorkspace  VariableName=Sysx_Out1  SaveFormat=Timeseries  SampleTime=-1
  y[k] To Workspace3 : ToWorkspace  VariableName=Sysx_Out2  SaveFormat=Timeseries  SampleTime=-1
  u_h : Outport
  wires:
  Sum4/1 -> u_h/1, Abs2/1
  Derivative/1 -> Mux4/2
  Mux4/1 -> CFGOC/1
  CFGOC/1 -> ta3_h/1, Integrator2/1
  Integrator2/1 -> ta4_h/1
  ta4_h/1 -> Sum4/2
  ta3_h/1 -> Sum4/1
  e_h/1 -> Abs/1, Derivative/1, Mux4/1
  Integrator3/1 -> y[k] To Workspace2/1
  Integrator4/1 -> y[k] To Workspace3/1
  Abs/1 -> Integrator3/1
  Abs2/1 -> Integrator4/1

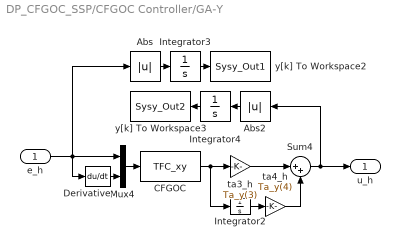
== system DP_CFGOC_SSP/CFGOC Controller/GA-Y ==
  e_h : Inport
  Abs : Abs  SaturateOnIntegerOverflow=off
  Abs2 : Abs  SaturateOnIntegerOverflow=off
  CFGOC : MATLABFcn  MATLABFcn=TFC_xy  OutputDimensions=1
  Derivative : Derivative
  Integrator2 : Integrator
  Integrator3 : Integrator
  Integrator4 : Integrator
  Mux4 : Mux  Inputs=2
  Sum4 : Sum  Inputs=|++  InputSameDT=on  SaturateOnIntegerOverflow=on  OutDataTypeStr=Inherit: Same as first input
  ta3_h : Gain  Gain=Ta_y(3)
  ta4_h : Gain  Gain=Ta_y(4)
  y[k] To Workspace2 : ToWorkspace  VariableName=Sysy_Out1  SaveFormat=Timeseries  SampleTime=-1
  y[k] To Workspace3 : ToWorkspace  VariableName=Sysy_Out2  SaveFormat=Timeseries  SampleTime=-1
  u_h : Outport
  wires:
  Sum4/1 -> u_h/1, Abs2/1
  Derivative/1 -> Mux4/2
  Mux4/1 -> CFGOC/1
  CFGOC/1 -> ta3_h/1, Integrator2/1
  Integrator2/1 -> ta4_h/1
  ta4_h/1 -> Sum4/2
  ta3_h/1 -> Sum4/1
  e_h/1 -> Abs/1, Derivative/1, Mux4/1
  Integrator3/1 -> y[k] To Workspace2/1
  Integrator4/1 -> y[k] To Workspace3/1
  Abs/1 -> Integrator3/1
  Abs2/1 -> Integrator4/1

== system DP_CFGOC_SSP/Subsystem/Current impact ==
  Current direction (deg) : Constant  Value=60
  Current speed (deg) : Constant  Value=0.5
  North-East current : Subsystem  AncestorBlock=marine_gnc/Environment/Current/North-East current
  Tau_current : Outport
  wires:
  Current speed (deg)/1 -> North-East current/2(V_c (m/s))
  Current direction (deg)/1 -> North-East current/1(beta_c (deg))
  North-East current/1(nu_c) -> Tau_current/1

== system DP_CFGOC_SSP/Subsystem/Noise impact ==
  "   " : simulink_extras/Transformations/Degrees to Radians
  Band-Limited White Noise : simulink/Sources/Band-Limited White Noise  Cov=[1]  Ts=0.1  seed=[23341]
  Linear 2nd-order wave spectrum1 : marine_gnc/Environment/Waves/Linear 2nd-order  wave spectrum  sigma=.5  w_0=1.2  lambda=0.1
  wave amplitude : Gain  Gain=3  SaturateOnIntegerOverflow=on  OutDataTypeStr=Inherit: Same as input  ParamDataTypeStr=Inherit: Same as input
  Tau_Noise : Outport
  wires:
  "   "/1 -> Tau_Noise/1
  Band-Limited White Noise/1 -> Linear 2nd-order wave spectrum1/1
  Linear 2nd-order wave spectrum1/1 -> wave amplitude/1
  wave amplitude/1 -> "   "/1

== system DP_CFGOC_SSP/Subsystem/Wave impact ==
  Location : Constant  Value=[0 0 0]
  Scope : Scope
  Wave velocitycalc : Subsystem  AncestorBlock=marine_gnc/Environment/Waves/Wave velocitycalc  mask(Wave velocitycalc){}
      mask help: Caclulates the wave-induced water velocity in NED coordinates and surface elevation Zeta at the point [x y z] in NED. The Waves bus generated by the Waves module is needed as input.
  Waves : marine_gnc/Environment/Waves/Waves  spectrum_type=ITTC  disp_flag=off  plot_spectrum=off  plot_realization=off  hs=0.8  omega_peak=0  psi_mean=0  gamma=-1  spread=2  depth=inf  nfreq=20  ndir=10  energylim=0.005  freq_cutoff=3  dir_cutoff=0  rand_seed=123  rand_freq=on  rand_dir=on  Zeta_a=0  Omega=0  Phase=0  Wavenum=0  Psi=0
  rad2deg : marine_gnc/Utilities/Math Operations/Unit Conversion  in=rad2deg
  wave direction : Display
  Tau_wave : Outport
  wires:
  Waves/1 -> Wave velocitycalc/2(Waves)
  Location/1 -> Wave velocitycalc/1("[x y z] NED")
  Wave velocitycalc/1(Zeta) -> Scope/1  "Wave elevation"
  Waves/2 -> rad2deg/1
  rad2deg/1 -> wave direction/1
  Wave velocitycalc/2(V_w NED) -> Tau_wave/1

== system DP_CFGOC_SSP/Subsystem/Wind impact ==
  psi : Inport
  Angle : Constant  Value=30
  Gain : Gain  Gain=0.5
  Mux : Mux  Inputs=3
  Vwind : Constant  Value=6
  Wind : Subsystem
  delay : TransferFcn  Denominator=[10 1]
  Tau_wind : Outport
  wires:
  Mux/1 -> Tau_wind/1
  Angle/1 -> Wind/2(thera)
  Vwind/1 -> Wind/1(Vw)
  Wind/1(Xwind) -> Mux/1
  Wind/2(Ywind) -> Mux/2
  Wind/3(Nwind) -> Mux/3
  psi/1 -> Gain/1
  Gain/1 -> delay/1
  delay/1 -> Wind/3(phi)

== system DP_CFGOC_SSP/Subsystem/Current impact/North-East current ==
  beta_c (deg) : Inport
  V_c (m/s) : Inport  Port=2
  Gain : Gain  Gain=pi/180
  Mux : Mux  Inputs=3
  Product : Product  RndMeth=Zero
  Product1 : Product  RndMeth=Zero
  cos : Trigonometry  Operator=cos
  sin : Trigonometry
  zero : Constant  Value=0
  nu_c : Outport
  wires:
  Mux/1 -> nu_c/1
  beta_c (deg)/1 -> Gain/1
  zero/1 -> Mux/3
  Product1/1 -> Mux/2
  Product/1 -> Mux/1
  sin/1 -> Product1/1
  V_c (m/s)/1 -> Product/2, Product1/2
  cos/1 -> Product/1
  Gain/1 -> cos/1, sin/1

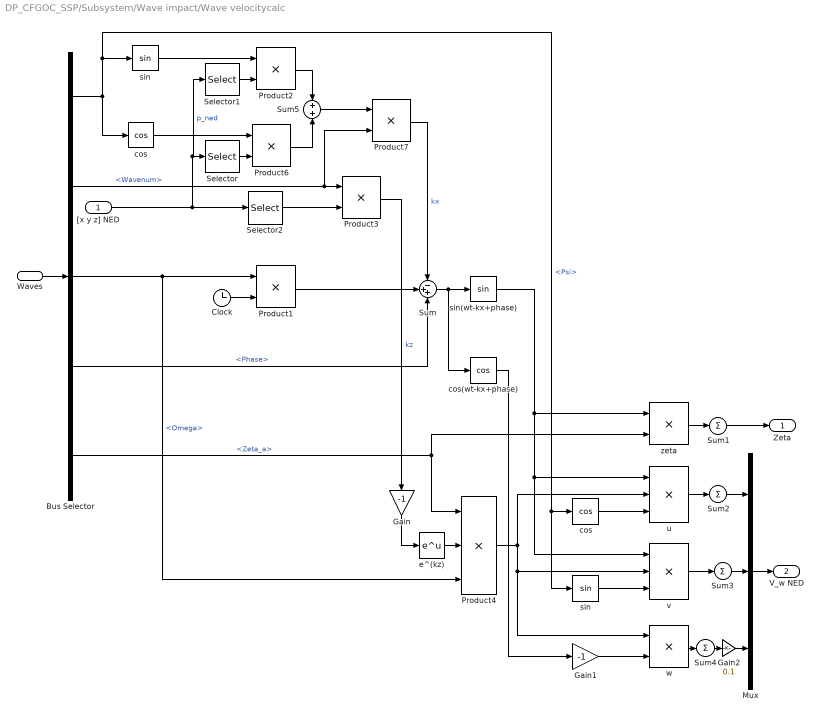
== system DP_CFGOC_SSP/Subsystem/Wave impact/Wave velocitycalc ==
  "[x y z] NED" : Inport
  Waves : Inport  Port=2
  Bus Selector : BusSelector  OutputSignals=Psi,Wavenum,Omega,Phase,Zeta_a
  Clock : Clock
  Gain : Gain  Gain=-1  SaturateOnIntegerOverflow=on  OutDataTypeStr=Inherit: Same as input  ParamDataTypeStr=Inherit: Same as input
  Gain1 : Gain  Gain=-1  SaturateOnIntegerOverflow=on  OutDataTypeStr=Inherit: Same as input  ParamDataTypeStr=Inherit: Same as input
  Gain2 : Gain  Gain=0.1  SaturateOnIntegerOverflow=on  OutDataTypeStr=Inherit: Same as input  ParamDataTypeStr=Inherit: Same as input
  Mux : Mux  Inputs=3
  Product{1..3,6..7} (5 alike) : Product  Inputs=**  SaturateOnIntegerOverflow=on  OutDataTypeStr=Inherit: Same as first input
  Product4 : Product  Inputs=3  SaturateOnIntegerOverflow=on  OutDataTypeStr=Inherit: Same as first input
  Selector : Selector  InputPortWidth=3  IndexOptions=Index vector (dialog)  Indices=1  OutputSizes=1
  Selector1 : Selector  InputPortWidth=3  IndexOptions=Index vector (dialog)  Indices=2  OutputSizes=1
  Selector2 : Selector  InputPortWidth=3  IndexOptions=Index vector (dialog)  Indices=3  OutputSizes=1
  Sum : Sum  Inputs=-++  SaturateOnIntegerOverflow=on
  Sum{1..4} (4 alike) : Sum  Inputs=1  SaturateOnIntegerOverflow=on
  Sum5 : Sum  SaturateOnIntegerOverflow=on
  cos : Trigonometry  Operator=cos
  "cos " : Trigonometry  Operator=cos
  cos(wt-kx+phase) : Trigonometry  Operator=cos
  e^(kz) : Math  SignedPower=on
  sin : Trigonometry
  "sin " : Trigonometry
  sin(wt-kx+phase) : Trigonometry
  u : Product  Inputs=***  SaturateOnIntegerOverflow=on  OutDataTypeStr=Inherit: Same as first input
  v : Product  Inputs=***  SaturateOnIntegerOverflow=on  OutDataTypeStr=Inherit: Same as first input
  w : Product  Inputs=**  SaturateOnIntegerOverflow=on  OutDataTypeStr=Inherit: Same as first input
  zeta : Product  Inputs=**  SaturateOnIntegerOverflow=on  OutDataTypeStr=Inherit: Same as first input
  Zeta : Outport
  V_w NED : Outport  Port=2
  wires:
  Clock/1 -> Product1/2
  Mux/1 -> V_w NED/1
  Sum3/1 -> Mux/2
  Sum2/1 -> Mux/1
  v/1 -> Sum3/1
  u/1 -> Sum2/1
  w/1 -> Sum4/1
  Sum1/1 -> Zeta/1
  Product3/1 -> Gain/1  "kz"
  Bus Selector/1 -> sin/1, "sin "/1, "cos "/1, cos/1  "<Psi>"
  Product1/1 -> Sum/2
  Sum/1 -> sin(wt-kx+phase)/1, cos(wt-kx+phase)/1
  sin(wt-kx+phase)/1 -> zeta/1, u/1, v/1
  zeta/1 -> Sum1/1
  Product7/1 -> Sum/1  "kx"
  e^(kz)/1 -> Product4/2
  Product4/1 -> u/2, v/2, w/1
  cos(wt-kx+phase)/1 -> Gain1/1
  Waves/1 -> Bus Selector/1
  Bus Selector/3 -> Product1/1, Product4/3  "<Omega>"
  Bus Selector/4 -> Sum/3  "<Phase>"
  Bus Selector/5 -> zeta/2, Product4/1  "<Zeta_a>"
  Gain/1 -> e^(kz)/1
  Bus Selector/2 -> Product7/2, Product3/1  "<Wavenum>"
  Selector/1 -> Product6/2
  cos/1 -> Product6/1
  Selector1/1 -> Product2/2
  sin/1 -> Product2/1
  Product2/1 -> Sum5/1
  Product6/1 -> Sum5/2
  Sum5/1 -> Product7/1
  "[x y z] NED"/1 -> Selector2/1, Selector1/1, Selector/1  "p_ned"
  Selector2/1 -> Product3/2
  "sin "/1 -> v/3
  "cos "/1 -> u/3
  Gain1/1 -> w/2
  Sum4/1 -> Gain2/1
  Gain2/1 -> Mux/3

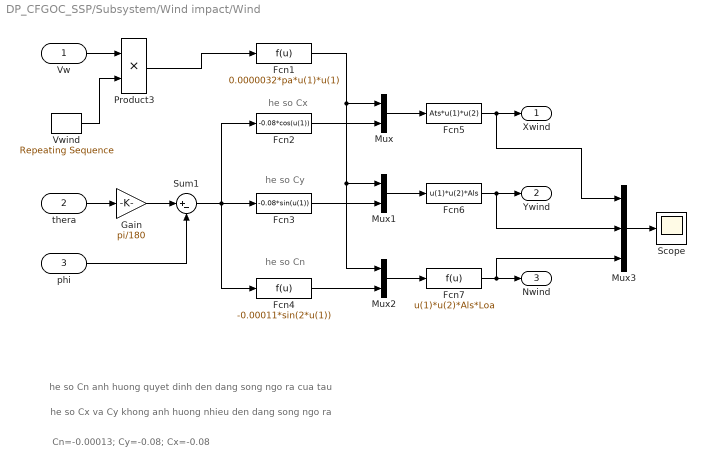
== system DP_CFGOC_SSP/Subsystem/Wind impact/Wind ==
  note: he so Cy
  note: he so Cn
  note: he so Cx
  note: he so Cn anh huong quyet dinh den dang song ngo ra cua tau
  note: he so Cx va Cy khong anh huong nhieu den dang song ngo ra
  note: Cn=-0.00013; Cy=-0.08; Cx=-0.08
  Vw : Inport
  thera : Inport  Port=2
  phi : Inport  Port=3
  Fcn1 : Fcn  Expr=0.0000032*pa*u(1)*u(1)
  Fcn2 : Fcn  Expr=-0.08*cos(u(1))
  Fcn3 : Fcn  Expr=-0.08*sin(u(1))
  Fcn4 : Fcn  Expr=-0.00011*sin(2*u(1))
  Fcn5 : Fcn  Expr=Ats*u(1)*u(2)
  Fcn6 : Fcn  Expr=u(1)*u(2)*Als
  Fcn7 : Fcn  Expr=u(1)*u(2)*Als*Loa
  Gain : Gain  Gain=pi/180
  Mux : Mux  Inputs=2
  Mux1 : Mux  Inputs=2
  Mux2 : Mux  Inputs=2
  Mux3 : Mux  Inputs=3
  Product3 : Product  RndMeth=Zero
  Scope : Scope
  Sum1 : Sum  Inputs=|+-
  Vwind : simulink/Sources/Repeating Sequence  rep_seq_t=[0 500 510 530 550 900 910 930 950 1100]  rep_seq_y=[0 0 1 1 0 0 1 1 0 0]
  Xwind : Outport
  Ywind : Outport  Port=2
  Nwind : Outport  Port=3
  wires:
  phi/1 -> Sum1/2
  Fcn1/1 -> Mux/1, Mux1/1, Mux2/1
  Mux/1 -> Fcn5/1
  Fcn5/1 -> Xwind/1, Mux3/1
  Mux1/1 -> Fcn6/1
  Mux2/1 -> Fcn7/1
  Fcn6/1 -> Ywind/1, Mux3/2
  Fcn7/1 -> Nwind/1, Mux3/3
  Gain/1 -> Sum1/1
  thera/1 -> Gain/1
  Sum1/1 -> Fcn3/1, Fcn2/1, Fcn4/1
  Fcn2/1 -> Mux/2
  Fcn3/1 -> Mux1/2
  Fcn4/1 -> Mux2/2
  Mux3/1 -> Scope/1
  Vw/1 -> Product3/1
  Product3/1 -> Fcn1/1
  Vwind/1 -> Product3/2
